simulink model "sim4"  (Simulink 9.0)
settings: Solver=ode15s  StartTime=0.0  StopTime=2  RelTol=1e-3  EnableMultiTasking=on
libraries: cstblocks x2, simulink x1
settings Model: Creator=gscorlet  LastModifiedBy=DEHAEZE
settings DataIOCC: LimitDataPoints=on  SignalLoggingSaveFormat=ModelDataLogs  Refine=10
settings OptimizationCC: BooleanDataType=off  ExpressionDepthLimit=2147483647  InitFltsAndDblsToZero=on
settings DebuggingCC: SaveWithParameterizedLinksMsg=none  SignalResolutionControl=TryResolveAllWithWarning  MultiTaskDSMMsg=warning  MultiTaskCondExecSysMsg=none  FcnCallInpInsideContextMsg=warning  StateNameClashWarn=warning  StrictBusMsg=None
settings HardwareCC: TargetUnknown=on
settings GRTTargetCC: GeneratePreprocessorConditionals=Disable all  CombineOutputUpdateFcns=off  GRTInterface=on

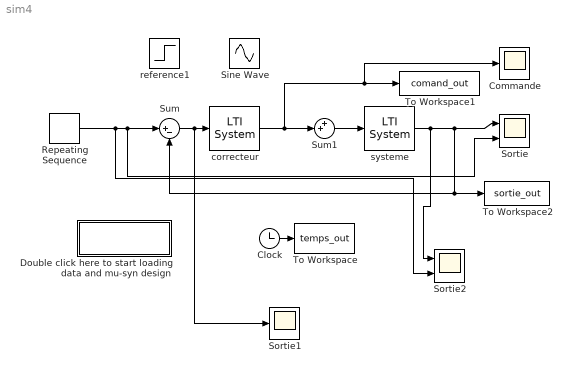
== system sim4 ==
  Clock : Clock
  Commande : Scope
  Double click here to start loading data and mu-syn design : Subsystem
      settings: OpenFcn=figure(FIG_SIM);subplot(211); plot(temps_out, sortie_out, 'r'); grid on; title('Sortie'); subplot(212); plot(temps_out, comand_out, 'r-'); title('Commande'); grid on;
      mask Display: disp('Plot figure')
  Repeating Sequence : simulink/Sources/Repeating Sequence  rep_seq_t=[0 0.05 0.1]  rep_seq_y=[0.06 -0.06 0.06]
  Sine Wave : Sin  Amplitude=0.05  Frequency=2*pi*50  SampleTime=0
  Sortie : Scope  NumInputPorts=2
  Sortie1 : Scope
  Sortie2 : Scope  NumInputPorts=2
  Sum : Sum  Inputs=|+-  SaturateOnIntegerOverflow=on  InputSameDT=on  OutDataTypeStr=Inherit: Same as first input
  Sum1 : Sum  Inputs=++|  SaturateOnIntegerOverflow=on  InputSameDT=on  OutDataTypeStr=Inherit: Same as first input
  To Workspace : ToWorkspace  VariableName=temps_out  SampleTime=-1
  To Workspace1 : ToWorkspace  VariableName=comand_out  SampleTime=-1
  To Workspace2 : ToWorkspace  VariableName=sortie_out  SampleTime=-1
  correcteur : cstblocks/LTI System  sys=ss_k  IC=0
  reference1 : Step  Time=0.5  SampleTime=0
  systeme : cstblocks/LTI System  sys=f_sys  IC=[]
  wires:
  Sum/1 -> correcteur/1, Sortie1/1
  Sum1/1 -> systeme/1
  correcteur/1 -> Sum1/2, To Workspace1/1, Commande/1
  Clock/1 -> To Workspace/1
  systeme/1 -> Sortie2/1, Sum/2, To Workspace2/1, Sortie/1
  Repeating Sequence/1 -> Sortie2/2, Sortie/2, Sum/1

== system sim4/Double click here to start loading data and mu-syn design ==
